simulink model "graficar_sintesis_analitica"  (R2024b)
settings: Solver=VariableStepAuto  StartTime=0.0  StopTime=10.0  RelTol=1e-3
settings Model: Creator=brandon  LastModifiedBy=brandon

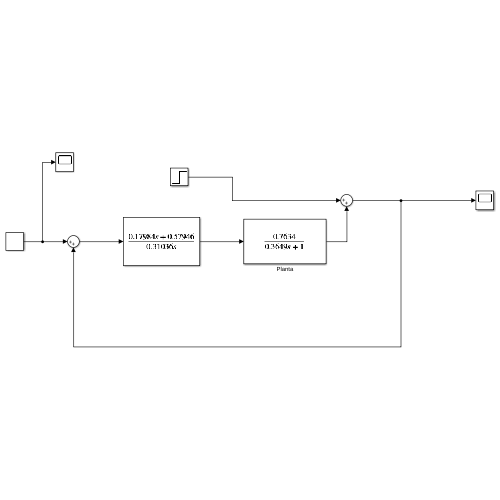
[thumbnail: Simulink's stored preview of the top-level diagram]
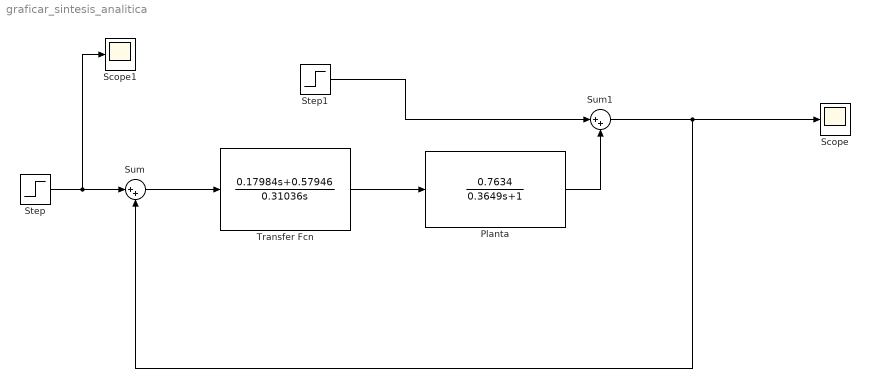
== system graficar_sintesis_analitica ==
  Planta : TransferFcn  Numerator=[0.7634]  Denominator=[0.3649 1]
  Scope : Scope
  Scope1 : Scope
  Step : Step  Time=22  Before=150  After=120  SampleTime=0
  Step1 : Step  Time=25  After=50  SampleTime=0.01
  Sum : Sum  Inputs=|++
  Sum1 : Sum  Inputs=|++
  Transfer Fcn : TransferFcn  Numerator=[0.17984 0.57946]  Denominator=[0.31036 0]
  wires:
  Step1/1 -> Sum1/1
  Planta/1 -> Sum1/2
  Transfer Fcn/1 -> Planta/1
  Sum/1 -> Transfer Fcn/1
  Step/1 -> Scope1/1, Sum/1
  Sum1/1 -> Scope/1, Sum/2
